simulink model "test_ffts"  (Simulink 6.2)
settings: Solver=ode45  StartTime=0.0  StopTime=300  RelTol=1e-3
undefined symbols (not defined in the file or in its folder): now
libraries: xbsIndex_r3 x1135, fft_library x1, simulink x1
(part 3 of 15)

== system test_ffts/r4_dit_fft ==
  a_in : Inport  Port=1  LatchInput=off
  b_in : Inport  Port=2  LatchInput=off
  c_in : Inport  Port=3  LatchInput=off
  d_in : Inport  Port=4  LatchInput=off
  sync_in : Inport  Port=5  LatchInput=off
  quadplex_bitrev : Subsystem  mask(Quadplex Bit Reverse Reorder){log2_size=4, n_bits=14}
      mask prompts: log2_size "Log2 Block Size"; n_bits "Number of Bits"
      mask help: Reorders the input sequences from normal order to bit reverse order (or vise versa).
      settings: AttributesFormatString=size = 16
      mask Help:
      | <pre>
      | Description::
      | 
      | Reorders the input sequences from normal order to bit reverse order (or vise versa).
      | 
      | Mask Parameters::
      | 
      | Log 2 Block Size (log2_size): The base-2 logarithm of the length of one complete input block.
      | This MUST be an integer because the current implementation requires that
      | the input block size MUST be a power of 2.  (aka "N")
      | 
      | Number of Bits (n_bits): Specifies the width of the real/imaginary components.
      | Width of each component is assumed equal.
      | </pre>
  quadplex_commutator : Subsystem  mask(Quadplex Commutator){log4_size=3, n_bits=14, use_bram=off}
      mask prompts: log4_size "Log4 Block Size"; n_bits "Bit Width"; use_bram "Use BRAM"
      mask help: The quadplex commutator performs a "quarter-blockwise" commutation of the four inputs. A "block" is 4^log4_size consecutive samples (i.e. always a power of 4). sync_in precedes the first data input sample by one clock cycle. Overall latency from sync_in to sync_out is 2^(log4_size)+2^(log4_size-1)+2.
      settings: AttributesFormatString=|
      | size = 64
      | 0/4 bram
      mask Help:
      | <pre>
      | Description::
      | 
      | The quadplex commutator performs a "quarter-blockwise" commutation of the four inputs.
      | A "block" is 4^log4_size consecutive samples (i.e. always a power of 4).
      | 
      | sync_in precedes the first data input sample by one clock cycle.
      | sync_out precedes the corresponding output sample by one clock cycle.
      | Overall latency from sync_in to sync_out is 2^(log4_size)+2^(log4_size-1)+2.
      | 
      | Mask Parameters::
      | 
      | Log4 Block Size (log4_size): The base-4 logarithm of the length of one complete input block.
      | This MUST be an integer because the current implementation requires that
      | the input block size MUST be a power of 4.  (aka "N")
      | 
      | Bit Width (n_bits): Specifies the width of the real/imaginary components.
      | Width of each component is assumed equal.
      | 
      | Use BRAM (use_bram): Check this checkbox to implement the internal delays using BRAM.
      | If unchecked, the internal delays will be implemented using SLR16 elements.
      | </pre>
  r4_dit_stage_1 : Subsystem  mask(Radix-4 DIT FFT Stage){n_stages=3, cur_stage=1, n_bits=8, bin_pt=7, shift=0, commutator_bram=off, twiddle_bram=off, n_bits_w=9, mult_latency=3, add_latency=1}
      mask prompts: n_stages "Total Stages (4^N points)"; cur_stage "Current Stage"; n_bits "Number of Bits In"; bin_pt "Binary Point In"; shift "Shift Bits"; commutator_bram "Use BRAM for Quadplex Commutator"; twiddle_bram "Use BRAM for Twiddle Coefficients"; n_bits_w "Twiddle Coefficient Bitwidth"; mult_latency "Multiplier Latency"; add_latency "Adder Latency"
      mask help: A radix-4 decimation-in-time Fast Fourier Transform stage.
      settings: AttributesFormatString=|
      | stage 1 of 3
      | delay slr
      | twiddle dist
      | shift 0
      mask Help:
      | <pre>
      | Description::
      | 
      | A radix-4 decimation-in-time Fast Fourier Transform stage.
      | 
      | This radix-4 decimation-in-time FFT stage is designed to be daisy chained together
      | to form a multi-stage FFT.  The resulting FFT will have (4^n_stages) points.
      | 
      | The four inputs to the chain are independent complex signals (e.g. A, B, C, and D).
      | 
      | The four outputs of the last stage of the chain are commuted such that the a_out signal is really
      | the first quarter of A's transform followed by the first quarter of B's transform, the first quarter
      | of C's transform and the first quarter of D's transform.  b_out is really the seconds quarter of
      | A's transform followed by the second quarter of B's transform and so on for the rest of b_out
      | as well as c_out and d_out.  Each quarter is in bit-reversed order.
      | 
      | If it is desired to have the four quarters of A's transform follow each other on the
      | same path (and so on for the transforms of B, C, and D), then a_out and b_out can
      | be fed through a quadplex_commutator with block size 4^n_stages.  This will result
      | in the four quarters of A's transform (or B's, C's, D's) being in sequential order,
      | but note that each quarter of A's transform will still remain in bit-reversed order
      | (i.e. each output is bit-reversed in quarterss; it is not bit reversed in its entirety).
      | 
      | The number of bits for each real and imaginary component grows by two through this stage.
      | If the input bit width is 17 or less, three embedded multipliers will be used per complex multiply.
      | If the input bit width is 18, four embedded multipliers will be used per complex multiply.
      | If the input bit width exceeds 18, then substantially more embedded multipliers will be used
      | per complex multiply.  Enabling "shifting" in some (or all) stages can limit the bit growth
      | to prevent this.
      | 
      | Mask Parameters::
      | 
      | Total Stages (n_stages):  The number of total stages in the FFT.
      | The FFT will have 4^n_stages points.
      | 
      | Current Stage (cur_stage):  The number of the current stage.  Note that stages are counted
      | from 1 to n_stages for DIT (i.e. cur_stage==1 for the first stage).
      | 
      | Number of Bits In (n_bits): Specifies the width of the real/imaginary components of ports
      | a_in and b_in.  Assumed equal for both components.  The real/imaginary components of
      | oorts a_out and b_out will be one bit wider.
      | 
      | Binary Point In (bin_pt): Specifies the binary point position of the real/imaginary
      | components of ports a_in and b_in.  Assumed equal for both components.
      | 
      | Shift Bits (shift): Specifies how many bits to shift (down) by.  A positive value causes
      | the specified number of least significant bits to be dropped.  Usually zero or positive values
      | are used to permit or limit bit growth, but negative values can be used to induce bit growth.
      | 
      | Use BRAM for Biplex Commutator (commutator_bram): Check this checkbox to implement
      | the biplex commutator using BRAM.  If unchecked, the biplex commutator will be implemented
      | using SLR16 elements (i.e. slices).
      | 
      | Use BRAM for Twiddle Coefficients (twiddle_bram): Check this checkbox to store twiddle
      | coefficients in BRAM.  If unchecked, the twiddle coefficients will be sored in distributed
      | memory (i.e. slices).
      | 
      | Twiddle Coefficient Bitwidth (n_bits_w): Specifies the width of the real/imaginary
      | components of the twiddle coefficients.  Assumed equal for both components.
      | 
      | Multiplier Latency (mult_latency): Latency to use for the underlying real multipliers.
      | 
      | Adder Latency (add_latency): Latency to use for the underlying real adders.
      | </pre>
  r4_dit_stage_2 : Subsystem  mask(Radix-4 DIT FFT Stage){n_stages=3, cur_stage=2, n_bits=10, bin_pt=7, shift=0, commutator_bram=off, twiddle_bram=off, n_bits_w=9, mult_latency=3, add_latency=1}
      mask prompts: n_stages "Total Stages (4^N points)"; cur_stage "Current Stage"; n_bits "Number of Bits In"; bin_pt "Binary Point In"; shift "Shift Bits"; commutator_bram "Use BRAM for Quadplex Commutator"; twiddle_bram "Use BRAM for Twiddle Coefficients"; n_bits_w "Twiddle Coefficient Bitwidth"; mult_latency "Multiplier Latency"; add_latency "Adder Latency"
      mask help: A radix-4 decimation-in-time Fast Fourier Transform stage.
      settings: AttributesFormatString=|
      | stage 2 of 3
      | delay slr
      | twiddle dist
      | shift 0
      mask Help:
      | <pre>
      | Description::
      | 
      | A radix-4 decimation-in-time Fast Fourier Transform stage.
      | 
      | This radix-4 decimation-in-time FFT stage is designed to be daisy chained together
      | to form a multi-stage FFT.  The resulting FFT will have (4^n_stages) points.
      | 
      | The four inputs to the chain are independent complex signals (e.g. A, B, C, and D).
      | 
      | The four outputs of the last stage of the chain are commuted such that the a_out signal is really
      | the first quarter of A's transform followed by the first quarter of B's transform, the first quarter
      | of C's transform and the first quarter of D's transform.  b_out is really the seconds quarter of
      | A's transform followed by the second quarter of B's transform and so on for the rest of b_out
      | as well as c_out and d_out.  Each quarter is in bit-reversed order.
      | 
      | If it is desired to have the four quarters of A's transform follow each other on the
      | same path (and so on for the transforms of B, C, and D), then a_out and b_out can
      | be fed through a quadplex_commutator with block size 4^n_stages.  This will result
      | in the four quarters of A's transform (or B's, C's, D's) being in sequential order,
      | but note that each quarter of A's transform will still remain in bit-reversed order
      | (i.e. each output is bit-reversed in quarterss; it is not bit reversed in its entirety).
      | 
      | The number of bits for each real and imaginary component grows by two through this stage.
      | If the input bit width is 17 or less, three embedded multipliers will be used per complex multiply.
      | If the input bit width is 18, four embedded multipliers will be used per complex multiply.
      | If the input bit width exceeds 18, then substantially more embedded multipliers will be used
      | per complex multiply.  Enabling "shifting" in some (or all) stages can limit the bit growth
      | to prevent this.
      | 
      | Mask Parameters::
      | 
      | Total Stages (n_stages):  The number of total stages in the FFT.
      | The FFT will have 4^n_stages points.
      | 
      | Current Stage (cur_stage):  The number of the current stage.  Note that stages are counted
      | from 1 to n_stages for DIT (i.e. cur_stage==1 for the first stage).
      | 
      | Number of Bits In (n_bits): Specifies the width of the real/imaginary components of ports
      | a_in and b_in.  Assumed equal for both components.  The real/imaginary components of
      | oorts a_out and b_out will be one bit wider.
      | 
      | Binary Point In (bin_pt): Specifies the binary point position of the real/imaginary
      | components of ports a_in and b_in.  Assumed equal for both components.
      | 
      | Shift Bits (shift): Specifies how many bits to shift (down) by.  A positive value causes
      | the specified number of least significant bits to be dropped.  Usually zero or positive values
      | are used to permit or limit bit growth, but negative values can be used to induce bit growth.
      | 
      | Use BRAM for Biplex Commutator (commutator_bram): Check this checkbox to implement
      | the biplex commutator using BRAM.  If unchecked, the biplex commutator will be implemented
      | using SLR16 elements (i.e. slices).
      | 
      | Use BRAM for Twiddle Coefficients (twiddle_bram): Check this checkbox to store twiddle
      | coefficients in BRAM.  If unchecked, the twiddle coefficients will be sored in distributed
      | memory (i.e. slices).
      | 
      | Twiddle Coefficient Bitwidth (n_bits_w): Specifies the width of the real/imaginary
      | components of the twiddle coefficients.  Assumed equal for both components.
      | 
      | Multiplier Latency (mult_latency): Latency to use for the underlying real multipliers.
      | 
      | Adder Latency (add_latency): Latency to use for the underlying real adders.
      | </pre>
  r4_dit_stage_3 : Subsystem  mask(Radix-4 DIT FFT Stage){n_stages=3, cur_stage=3, n_bits=12, bin_pt=7, shift=0, commutator_bram=off, twiddle_bram=off, n_bits_w=9, mult_latency=3, add_latency=1}
      mask prompts: n_stages "Total Stages (4^N points)"; cur_stage "Current Stage"; n_bits "Number of Bits In"; bin_pt "Binary Point In"; shift "Shift Bits"; commutator_bram "Use BRAM for Quadplex Commutator"; twiddle_bram "Use BRAM for Twiddle Coefficients"; n_bits_w "Twiddle Coefficient Bitwidth"; mult_latency "Multiplier Latency"; add_latency "Adder Latency"
      mask help: A radix-4 decimation-in-time Fast Fourier Transform stage.
      settings: AttributesFormatString=|
      | stage 3 of 3
      | delay slr
      | twiddle dist
      | shift 0
      mask Help:
      | <pre>
      | Description::
      | 
      | A radix-4 decimation-in-time Fast Fourier Transform stage.
      | 
      | This radix-4 decimation-in-time FFT stage is designed to be daisy chained together
      | to form a multi-stage FFT.  The resulting FFT will have (4^n_stages) points.
      | 
      | The four inputs to the chain are independent complex signals (e.g. A, B, C, and D).
      | 
      | The four outputs of the last stage of the chain are commuted such that the a_out signal is really
      | the first quarter of A's transform followed by the first quarter of B's transform, the first quarter
      | of C's transform and the first quarter of D's transform.  b_out is really the seconds quarter of
      | A's transform followed by the second quarter of B's transform and so on for the rest of b_out
      | as well as c_out and d_out.  Each quarter is in bit-reversed order.
      | 
      | If it is desired to have the four quarters of A's transform follow each other on the
      | same path (and so on for the transforms of B, C, and D), then a_out and b_out can
      | be fed through a quadplex_commutator with block size 4^n_stages.  This will result
      | in the four quarters of A's transform (or B's, C's, D's) being in sequential order,
      | but note that each quarter of A's transform will still remain in bit-reversed order
      | (i.e. each output is bit-reversed in quarterss; it is not bit reversed in its entirety).
      | 
      | The number of bits for each real and imaginary component grows by two through this stage.
      | If the input bit width is 17 or less, three embedded multipliers will be used per complex multiply.
      | If the input bit width is 18, four embedded multipliers will be used per complex multiply.
      | If the input bit width exceeds 18, then substantially more embedded multipliers will be used
      | per complex multiply.  Enabling "shifting" in some (or all) stages can limit the bit growth
      | to prevent this.
      | 
      | Mask Parameters::
      | 
      | Total Stages (n_stages):  The number of total stages in the FFT.
      | The FFT will have 4^n_stages points.
      | 
      | Current Stage (cur_stage):  The number of the current stage.  Note that stages are counted
      | from 1 to n_stages for DIT (i.e. cur_stage==1 for the first stage).
      | 
      | Number of Bits In (n_bits): Specifies the width of the real/imaginary components of ports
      | a_in and b_in.  Assumed equal for both components.  The real/imaginary components of
      | oorts a_out and b_out will be one bit wider.
      | 
      | Binary Point In (bin_pt): Specifies the binary point position of the real/imaginary
      | components of ports a_in and b_in.  Assumed equal for both components.
      | 
      | Shift Bits (shift): Specifies how many bits to shift (down) by.  A positive value causes
      | the specified number of least significant bits to be dropped.  Usually zero or positive values
      | are used to permit or limit bit growth, but negative values can be used to induce bit growth.
      | 
      | Use BRAM for Biplex Commutator (commutator_bram): Check this checkbox to implement
      | the biplex commutator using BRAM.  If unchecked, the biplex commutator will be implemented
      | using SLR16 elements (i.e. slices).
      | 
      | Use BRAM for Twiddle Coefficients (twiddle_bram): Check this checkbox to store twiddle
      | coefficients in BRAM.  If unchecked, the twiddle coefficients will be sored in distributed
      | memory (i.e. slices).
      | 
      | Twiddle Coefficient Bitwidth (n_bits_w): Specifies the width of the real/imaginary
      | components of the twiddle coefficients.  Assumed equal for both components.
      | 
      | Multiplier Latency (mult_latency): Latency to use for the underlying real multipliers.
      | 
      | Adder Latency (add_latency): Latency to use for the underlying real adders.
      | </pre>
  a_out : Outport
  b_out : Outport  Port=2
  c_out : Outport  Port=3
  d_out : Outport  Port=4
  sync_out : Outport  Port=5
  wires:
  a_in/1 -> r4_dit_stage_1/1(a_in)
  b_in/1 -> r4_dit_stage_1/2(b_in)
  c_in/1 -> r4_dit_stage_1/3(c_in)
  d_in/1 -> r4_dit_stage_1/4(d_in)
  sync_in/1 -> r4_dit_stage_1/5(sync_in)
  r4_dit_stage_1/1(a_out) -> r4_dit_stage_2/1(a_in)
  r4_dit_stage_1/2(b_out) -> r4_dit_stage_2/2(b_in)
  r4_dit_stage_1/3(c_out) -> r4_dit_stage_2/3(c_in)
  r4_dit_stage_1/4(d_out) -> r4_dit_stage_2/4(d_in)
  r4_dit_stage_1/5(sync_out) -> r4_dit_stage_2/5(sync_in)
  r4_dit_stage_2/1(a_out) -> r4_dit_stage_3/1(a_in)
  r4_dit_stage_2/2(b_out) -> r4_dit_stage_3/2(b_in)
  r4_dit_stage_2/3(c_out) -> r4_dit_stage_3/3(c_in)
  r4_dit_stage_2/4(d_out) -> r4_dit_stage_3/4(d_in)
  r4_dit_stage_2/5(sync_out) -> r4_dit_stage_3/5(sync_in)
  r4_dit_stage_3/1(a_out) -> quadplex_commutator/1(a)
  r4_dit_stage_3/3(c_out) -> quadplex_commutator/2(b)
  r4_dit_stage_3/2(b_out) -> quadplex_commutator/3(c)
  r4_dit_stage_3/4(d_out) -> quadplex_commutator/4(d)
  r4_dit_stage_3/5(sync_out) -> quadplex_commutator/5(sync_in)
  quadplex_commutator/1(abcd0) -> quadplex_bitrev/1(a_in)
  quadplex_commutator/2(abcd1) -> quadplex_bitrev/2(b_in)
  quadplex_commutator/3(abcd2) -> quadplex_bitrev/3(c_in)
  quadplex_commutator/4(abcd3) -> quadplex_bitrev/4(d_in)
  quadplex_commutator/5(sync_out) -> quadplex_bitrev/5(sync_in)
  quadplex_bitrev/1(a_out) -> a_out/1
  quadplex_bitrev/2(b_out) -> b_out/1
  quadplex_bitrev/3(c_out) -> c_out/1
  quadplex_bitrev/4(d_out) -> d_out/1
  quadplex_bitrev/5(sync_out) -> sync_out/1

== system test_ffts/ri_to_c ==
  re : Inport  Port=1  LatchInput=off
  im : Inport  Port=2  LatchInput=off
  concat : xbsIndex_r3/Concat  num_inputs=2  explicit_period=off  period=1  dbl_ovrd=off
  force_im : xbsIndex_r3/Reinterpret  force_arith_type=on  arith_type=Unsigned  force_bin_pt=on  bin_pt=0  force_valid=on
  force_re : xbsIndex_r3/Reinterpret  force_arith_type=on  arith_type=Unsigned  force_bin_pt=on  bin_pt=0  force_valid=on
  c : Outport
  wires:
  force_re/1 -> concat/1
  force_im/1 -> concat/2
  re/1 -> force_re/1
  concat/1 -> c/1
  im/1 -> force_im/1

== system test_ffts/ri_to_c1 ==
  re : Inport  Port=1  LatchInput=off
  im : Inport  Port=2  LatchInput=off
  concat : xbsIndex_r3/Concat  num_inputs=2  explicit_period=off  period=1  dbl_ovrd=off
  force_im : xbsIndex_r3/Reinterpret  force_arith_type=on  arith_type=Unsigned  force_bin_pt=on  bin_pt=0  force_valid=on
  force_re : xbsIndex_r3/Reinterpret  force_arith_type=on  arith_type=Unsigned  force_bin_pt=on  bin_pt=0  force_valid=on
  c : Outport
  wires:
  im/1 -> force_im/1
  concat/1 -> c/1
  re/1 -> force_re/1
  force_im/1 -> concat/2
  force_re/1 -> concat/1

== system test_ffts/ri_to_c2 ==
  re : Inport  Port=1  LatchInput=off
  im : Inport  Port=2  LatchInput=off
  concat : xbsIndex_r3/Concat  num_inputs=2  explicit_period=off  period=1  dbl_ovrd=off
  force_im : xbsIndex_r3/Reinterpret  force_arith_type=on  arith_type=Unsigned  force_bin_pt=on  bin_pt=0  force_valid=on
  force_re : xbsIndex_r3/Reinterpret  force_arith_type=on  arith_type=Unsigned  force_bin_pt=on  bin_pt=0  force_valid=on
  c : Outport
  wires:
  im/1 -> force_im/1
  concat/1 -> c/1
  re/1 -> force_re/1
  force_im/1 -> concat/2
  force_re/1 -> concat/1

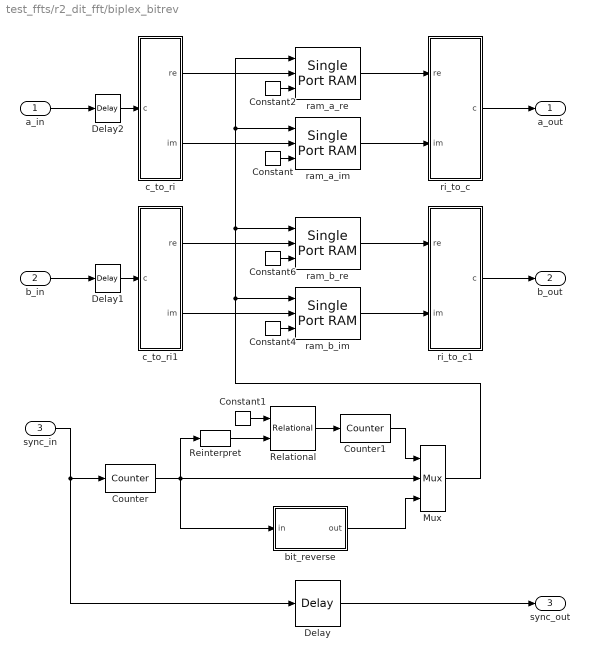
== system test_ffts/r2_dit_fft/biplex_bitrev ==
  a_in : Inport  Port=1  LatchInput=off
  b_in : Inport  Port=2  LatchInput=off
  sync_in : Inport  Port=3  LatchInput=off
  Constant{,2,4,6} (4 alike) : xbsIndex_r3/Constant  const=1  equ=P=C  arith_type=Boolean  n_bits=1  bin_pt=0  opselect=C  inp2=PCIN>>17  opr=+  inp1=P  carry=CIN  iostate=0  explicit_period=on  period=1  dbl_ovrd=off
  Constant1 : xbsIndex_r3/Constant  const=-1  equ=P=C  arith_type="Signed  (2's comp)"  n_bits=1  bin_pt=0  opselect=C  inp2=PCIN>>17  opr=+  inp1=P  carry=CIN  iostate=0  explicit_period=on  period=1  dbl_ovrd=off
  Counter : xbsIndex_r3/Counter  cnt_type=Free Running  n_bits=5  bin_pt=0  arith_type=Unsigned  start_count=0  cnt_to=Inf  cnt_by_val=1  operation=Up  explicit_period=off  period=1  load_pin=off  rst=on  en=off  dbl_ovrd=off  show_param=off  use_rpm=on  gen_core=off
      settings: xl_area=[0, 0, 0, 0, 0, 0, 0]
  Counter1 : xbsIndex_r3/Counter  cnt_type=Free Running  n_bits=1  bin_pt=0  arith_type=Unsigned  start_count=0  cnt_to=Inf  cnt_by_val=1  operation=Up  explicit_period=off  period=1  load_pin=off  rst=off  en=on  dbl_ovrd=off  show_param=off  use_rpm=on  gen_core=off
      settings: xl_area=[0, 0, 0, 0, 0, 0, 0]
  Delay : xbsIndex_r3/Delay  latency=34  reg_retiming=off  explicit_period=off  period=1  en=off  accept_only_valid=off  init_zero=on  dbl_ovrd=off  show_param=off
      settings: xl_area=[0, 0, 0, 0, 0, 0, 0]
  Delay1 : xbsIndex_r3/Delay  latency=1  reg_retiming=off  explicit_period=off  period=1  en=off  accept_only_valid=off  init_zero=on  dbl_ovrd=off  show_param=off
      settings: xl_area=[0, 0, 0, 0, 0, 0, 0]
  Delay2 : xbsIndex_r3/Delay  latency=1  reg_retiming=off  explicit_period=off  period=1  en=off  accept_only_valid=off  init_zero=on  dbl_ovrd=off  show_param=off
      settings: xl_area=[0, 0, 0, 0, 0, 0, 0]
  Mux : xbsIndex_r3/Mux  inputs=2  precision=Full  arith_type="Signed  (2's comp)"  n_bits=8  bin_pt=2  quantization=Truncate  overflow=Wrap  latency=1  explicit_period=off  period=1  en=off  dbl_ovrd=off  show_param=off  mux_type=off  use_rpm=off  gen_core=off
      settings: xl_area=[0, 0, 0, 0, 0, 0, 0]
  Reinterpret : xbsIndex_r3/Reinterpret  force_arith_type=on  arith_type="Signed  (2's comp)"  force_bin_pt=off  bin_pt=0  force_valid=on
  Relational : xbsIndex_r3/Relational  mode=a=b  latency=1  explicit_period=off  period=1  en=off  dbl_ovrd=off  show_param=off
      settings: xl_area=[0, 0, 0, 0, 0, 0, 0]
  bit_reverse : Subsystem  mask(Bit Reversal){n_bits=5}
      mask prompts: n_bits "Number of Bits"
      mask help: Reverses the bit order of the input. Input must be unsigned with binary point at position 0. Costs nothing in hardware.
      settings: AttributesFormatString=5 bits
      mask Help:
      | <pre>
      | Description::
      | 
      | Reverses the bit order of the input.
      | 
      | Input must be unsigned with binary point at position 0.
      | 
      | Costs nothing in hardware.
      | 
      | Mask Parameters::
      | 
      | Number of Bits (n_bits): Specifies the width of the input.
      | </pre>
  c_to_ri : Subsystem  mask(Complex to Real-Imag){n_bits=14, bin_pt=0}
      mask prompts: n_bits "Bit Width"; bin_pt "Binary Point"
      mask help: Outputs real and imaginary components of a complex input.
      settings: AttributesFormatString=14_0 r/i
      mask Help:
      | <pre>
      | Description::
      | 
      | Outputs real and imaginary components of a complex input.
      | Useful for simplifying interconnects.
      | See also: Real-Imag to Complex (ri_to_c)
      | 
      | Mask Parameters::
      | 
      | Bit Width (n_bits): Specifies the width of the real/imaginary components.
      | Assumed equal for both components.
      | 
      | Binary Point (bin_pt): Specifies the binary point location in the real/imaginary components.
      | Assumed equal for both components.
      | </pre>
  c_to_ri1 : Subsystem  mask(Complex to Real-Imag){n_bits=14, bin_pt=0}
      mask prompts: n_bits "Bit Width"; bin_pt "Binary Point"
      mask help: Outputs real and imaginary components of a complex input.
      settings: AttributesFormatString=14_0 r/i
      mask Help:
      | <pre>
      | Description::
      | 
      | Outputs real and imaginary components of a complex input.
      | Useful for simplifying interconnects.
      | See also: Real-Imag to Complex (ri_to_c)
      | 
      | Mask Parameters::
      | 
      | Bit Width (n_bits): Specifies the width of the real/imaginary components.
      | Assumed equal for both components.
      | 
      | Binary Point (bin_pt): Specifies the binary point location in the real/imaginary components.
      | Assumed equal for both components.
      | </pre>
  ram_a_im : xbsIndex_r3/Single Port RAM  depth=32  initVector=0  write_mode=Read Before Write  latency=1  init_zero=on  explicit_period=off  period=1  rst=off  init_reg=0  en=off  dbl_ovrd=off  show_param=on  distributed_mem=off  use_rpm=off  gen_core=off
      settings: xl_area=[0, 0, 0, 0, 0, 0, 0]
  ram_a_re : xbsIndex_r3/Single Port RAM  depth=32  initVector=0  write_mode=Read Before Write  latency=1  init_zero=on  explicit_period=off  period=1  rst=off  init_reg=0  en=off  dbl_ovrd=off  show_param=on  distributed_mem=off  use_rpm=off  gen_core=off
      settings: xl_area=[0, 0, 0, 0, 0, 0, 0]
  ram_b_im : xbsIndex_r3/Single Port RAM  depth=32  initVector=0  write_mode=Read Before Write  latency=1  init_zero=on  explicit_period=off  period=1  rst=off  init_reg=0  en=off  dbl_ovrd=off  show_param=on  distributed_mem=off  use_rpm=off  gen_core=off
      settings: xl_area=[0, 0, 0, 0, 0, 0, 0]
  ram_b_re : xbsIndex_r3/Single Port RAM  depth=32  initVector=0  write_mode=Read Before Write  latency=1  init_zero=on  explicit_period=off  period=1  rst=off  init_reg=0  en=off  dbl_ovrd=off  show_param=on  distributed_mem=off  use_rpm=off  gen_core=off
      settings: xl_area=[0, 0, 0, 0, 0, 0, 0]
  ri_to_c : Subsystem
      mask Type: Real-Imag to Complex
      mask Description: Concatenates real and imaginary inputs into a complex output.
      mask Help:
      | <pre>
      | Description::
      | 
      | Concatenates a real and imaginary input into a complex output.
      | Useful for simplifying interconnects.
      | See also: Complex to Real-Imag (c_to_ri)
      | 
      | Mask Parameters::
      | 
      | (N/A)
      | </pre>
  ri_to_c1 : Subsystem
      mask Type: Real-Imag to Complex
      mask Description: Concatenates real and imaginary inputs into a complex output.
      mask Help:
      | <pre>
      | Description::
      | 
      | Concatenates a real and imaginary input into a complex output.
      | Useful for simplifying interconnects.
      | See also: Complex to Real-Imag (c_to_ri)
      | 
      | Mask Parameters::
      | 
      | (N/A)
      | </pre>
  a_out : Outport
  b_out : Outport  Port=2
  sync_out : Outport  Port=3
  wires:
  Reinterpret/1 -> Relational/2
  Relational/1 -> Counter1/1
  Constant1/1 -> Relational/1
  Counter1/1 -> Mux/1
  Counter/1 -> Reinterpret/1, Mux/2, bit_reverse/1(in)
  Constant6/1 -> ram_b_re/3
  Constant4/1 -> ram_b_im/3
  Constant2/1 -> ram_a_re/3
  Constant/1 -> ram_a_im/3
  Delay/1 -> sync_out/1
  Mux/1 -> ram_b_im/1, ram_b_re/1, ram_a_im/1, ram_a_re/1
  bit_reverse/1(out) -> Mux/3
  b_in/1 -> Delay1/1
  a_in/1 -> Delay2/1
  c_to_ri1/2(im) -> ram_b_im/2
  c_to_ri1/1(re) -> ram_b_re/2
  c_to_ri/2(im) -> ram_a_im/2
  c_to_ri/1(re) -> ram_a_re/2
  ri_to_c1/1(c) -> b_out/1
  ri_to_c/1(c) -> a_out/1
  ram_b_im/1 -> ri_to_c1/2(im)
  ram_b_re/1 -> ri_to_c1/1(re)
  ram_a_im/1 -> ri_to_c/2(im)
  ram_a_re/1 -> ri_to_c/1(re)
  sync_in/1 -> Delay/1, Counter/1
  Delay1/1 -> c_to_ri1/1(c)
  Delay2/1 -> c_to_ri/1(c)

== system test_ffts/r2_dit_fft/biplex_commutator ==
  AloAhi : Inport  Port=1  LatchInput=off
  BloBhi : Inport  Port=2  LatchInput=off
  sync_in : Inport  Port=3  LatchInput=off
  Counter : xbsIndex_r3/Counter  cnt_type=Free Running  n_bits=6  bin_pt=0  arith_type=Unsigned  start_count=0  cnt_to=Inf  cnt_by_val=1  operation=Up  explicit_period=off  period=1  load_pin=off  rst=on  en=off  dbl_ovrd=off  show_param=off  use_rpm=on  gen_core=off
      settings: xl_area=[0, 0, 0, 0, 0, 0, 0]
  Delay : xbsIndex_r3/Delay  latency=33  reg_retiming=off  explicit_period=off  period=1  en=off  accept_only_valid=off  init_zero=on  dbl_ovrd=off  show_param=off
      settings: xl_area=[0, 0, 0, 0, 0, 0, 0]
  Mux : xbsIndex_r3/Mux  inputs=2  precision=Full  arith_type="Signed  (2's comp)"  n_bits=8  bin_pt=2  quantization=Truncate  overflow=Wrap  latency=1  explicit_period=off  period=1  en=off  dbl_ovrd=off  show_param=off  mux_type=off  use_rpm=off  gen_core=off
      settings: xl_area=[0, 0, 0, 0, 0, 0, 0]
  Mux1 : xbsIndex_r3/Mux  inputs=2  precision=Full  arith_type="Signed  (2's comp)"  n_bits=8  bin_pt=2  quantization=Truncate  overflow=Wrap  latency=1  explicit_period=off  period=1  en=off  dbl_ovrd=off  show_param=on  mux_type=off  use_rpm=off  gen_core=off
      settings: xl_area=[0, 0, 0, 0, 0, 0, 0]
  delay_b : Subsystem  mask(Complex Delay){delay_depth=32, n_bits=14, use_bram=on}
      mask prompts: delay_depth "Delay Depth"; n_bits "Bit Width"; use_bram "Use BRAM"
      mask help: A delay block that treats its input as complex, splits it into real and imaginary components, delays each component by a specified amount, and then re-joins them into a complex output. The underlying storage is user-selectable (either BRAM or SLR16 elements).
      settings: AttributesFormatString=|
      | depth = 32
      | delay bram
      mask Help:
      | <pre>
      | Description::
      | 
      | A delay block that treats its input as complex, splits it into real and imaginary components,
      | delays each component by a specified amount, and then re-joins them into a complex
      | output.  The underlying storage is user-selectable (either BRAM or SLR16 elements).
      | 
      | Mask Parameters::
      | 
      | Delay Depth (delay_depth): The length of the delay.
      | 
      | Bit Width (n_bits): Specifies the width of the real/imaginary components.
      | Width of each component is assumed equal.
      | 
      | Use BRAM (use_bram): Check this checkbox to implement the delay using BRAM.
      | If unchecked, the delay will be implemented using SLR16 elements.
      | </pre>
  delay_lo : Subsystem  mask(Complex Delay){delay_depth=32, n_bits=14, use_bram=on}
      mask prompts: delay_depth "Delay Depth"; n_bits "Bit Width"; use_bram "Use BRAM"
      mask help: A delay block that treats its input as complex, splits it into real and imaginary components, delays each component by a specified amount, and then re-joins them into a complex output. The underlying storage is user-selectable (either BRAM or SLR16 elements).
      settings: AttributesFormatString=|
      | depth = 32
      | delay bram
      mask Help:
      | <pre>
      | Description::
      | 
      | A delay block that treats its input as complex, splits it into real and imaginary components,
      | delays each component by a specified amount, and then re-joins them into a complex
      | output.  The underlying storage is user-selectable (either BRAM or SLR16 elements).
      | 
      | Mask Parameters::
      | 
      | Delay Depth (delay_depth): The length of the delay.
      | 
      | Bit Width (n_bits): Specifies the width of the real/imaginary components.
      | Width of each component is assumed equal.
      | 
      | Use BRAM (use_bram): Check this checkbox to implement the delay using BRAM.
      | If unchecked, the delay will be implemented using SLR16 elements.
      | </pre>
  top_bit : xbsIndex_r3/Slice  mode=Upper Bit Location + Width  nbits=1  bit1=0  base1=MSB of Input  bit0=0  base0=LSB of Input  boolean_output=off  explicit_period=off  period=1  dbl_ovrd=off
  AloBlo : Outport
  AhiBhi : Outport  Port=2
  sync_out : Outport  Port=3
  wires:
  Delay/1 -> sync_out/1
  delay_lo/1(out) -> AloBlo/1
  Mux/1 -> delay_lo/1(in)
  delay_b/1(out) -> Mux/3, Mux1/2
  BloBhi/1 -> delay_b/1(in)
  Mux1/1 -> AhiBhi/1
  AloAhi/1 -> Mux1/3, Mux/2
  top_bit/1 -> Mux/1, Mux1/1
  Counter/1 -> top_bit/1
  sync_in/1 -> Delay/1, Counter/1

== system test_ffts/r2_dit_fft/r2_dit_stage_1 ==
  a_in : Inport  Port=1  LatchInput=off
  b_in : Inport  Port=2  LatchInput=off
  sync_in : Inport  Port=3  LatchInput=off
  biplex_commutator : Subsystem  mask(Biplex Commutator){log2_size=6, n_bits=8, use_bram=off}
      mask prompts: log2_size "Log2 Block Size"; n_bits "Bit Width"; use_bram "Use BRAM"
      mask help: The biplex commutator commutes the first half of the BloBhi input "block" with the last half of the AloAhi input "block". A "block" is 2^log2_size consecutive samples (i.e. always a power of 2). sync_in precedes the first data input sample by one clock cycle. Overall latency from sync_in to sync_out is 2^(log2_size-1)+1.
      settings: AttributesFormatString=|
      | size = 64
      | delay slr
      mask Help:
      | <pre>
      | Description::
      | 
      | The biplex commutator commutes the first half of the BloBhi input "block"  with the last half
      | of the AloAhi input "block".  A "block" is 2^log2_size consecutive samples (i.e. always a
      | power of 2).
      | 
      | sync_in precedes the first data input sample by one clock cycle.
      | sync_out precedes the corresponding output sample by one clock cycle.
      | Overall latency from sync_in to sync_out is 2^(N-1)+1.
      | 
      | Mask Parameters::
      | 
      | Log 2 Block Size (log2_size): The base-2 logarithm of the length of one complete input block.
      | This MUST be an integer because the current implementation requires that
      | the input block size MUST be a power of 2.  (aka "N")
      | 
      | Bit Width (n_bits): Specifies the width of the real/imaginary components.
      | Width of each component is assumed equal.
      | 
      | Use BRAM (use_bram): Check this checkbox to implement the internal delays using BRAM.
      | If unchecked, the internal delays will be implemented using SLR16 elements.
      | </pre>
  r2_butterfly : Subsystem  mask(Radix-2 Butterfly){n_bits=8, shift=0, quantization=Truncate, add_latency=1}
      mask prompts: n_bits "Bit Width In"; shift "Shift Bits"; add_latency "Adder Latency"
      mask help: The radix-2 butterfly produces a+b and a-b outputs for a and b inputs.
      settings: AttributesFormatString=shift 0
      mask Help:
      | <pre>
      | Description::
      | 
      | The radix-2 butterfly produces a+b and a-b outputs for a and b inputs.
      | The outputs are one bit wider than the inputs.
      | The output precision (i.e. the number of fractional bits) stays the same.
      | 
      | Mask Parameters::
      | 
      | Bit Width In (n_bits): Specifies the width of the real/imaginary components.
      | Width of each component is assumed equal.
      | 
      | Shift Bits (shift): Specifies how many bits to shift (down) by.  A positive value causes
      | the specified number of least significant bits to be dropped.  Usually zero or positive values
      | are used to permit or limit bit growth, but negative values can be used to induce bit growth.
      | 
      | Quantization (quantization): Specifies quantization handling (when shift bits > 0).
      | 
      | Adder Latency (add_latency): Latency to use for the underlying real adders.
      | </pre>
      mask StyleString: edit,edit,popup(Truncate|Round  (unbiased: +/- Inf)|Round  (unbiased: Even Values)),edit
  r2_twiddle : Subsystem
      mask Type: Radix-2 Stage-1 Twiddle Stage
      mask Description: A stage-1 twiddle stage for radix-2 Fast Fourier Transforms. Since there are no twiddles in stage 1 of an FFT, this is just a dummy placeholder block that passes its inputs through to its outputs.    Since it is a no-op, its use is completely optional.
      mask Help:
      | <pre>
      | Description::
      | 
      | A stage-1 twiddle stage for radix-2 Fast Fourier Transforms.
      | 
      | Since there are no twiddles in stage 1 of an FFT, this is just a dummy placeholder
      | block that passes its inputs through to its outputs.
      | 
      | Since it is a no-op, its use is completely optional.
      | 
      | Note that stages are counted from 1 to n_stages for DIT (i.e. cur_stage==1 for the first stage)
      | and n_stages to 1for DIF (i.e. cur_stage==1 for the last stage).  Therefore, this block, if used,
      | should be the first twiddle stage of a DIT FFT or the last twiddle stage of a DIF FFT.
      | 
      | Mask Parameters::
      | 
      | (N/A)
  a_out : Outport
  b_out : Outport  Port=2
  sync_out : Outport  Port=3
  wires:
  r2_butterfly/3(sync_out) -> sync_out/1
  r2_butterfly/2(a-b) -> b_out/1
  r2_butterfly/1(a+b) -> a_out/1
  sync_in/1 -> biplex_commutator/3(sync_in)
  b_in/1 -> biplex_commutator/2(BloBhi)
  a_in/1 -> biplex_commutator/1(AloAhi)
  biplex_commutator/3(sync_out) -> r2_twiddle/3(sync_in)
  biplex_commutator/2(AhiBhi) -> r2_twiddle/2(b_in)
  biplex_commutator/1(AloBlo) -> r2_twiddle/1(a_in)
  r2_twiddle/1(a_out) -> r2_butterfly/1(a)
  r2_twiddle/2(b_out) -> r2_butterfly/2(b)
  r2_twiddle/3(sync_out) -> r2_butterfly/3(sync_in)

== system test_ffts/r2_dit_fft/r2_dit_stage_2 ==
  a_in : Inport  Port=1  LatchInput=off
  b_in : Inport  Port=2  LatchInput=off
  sync_in : Inport  Port=3  LatchInput=off
  biplex_commutator : Subsystem  mask(Biplex Commutator){log2_size=5, n_bits=9, use_bram=off}
      mask prompts: log2_size "Log2 Block Size"; n_bits "Bit Width"; use_bram "Use BRAM"
      mask help: The biplex commutator commutes the first half of the BloBhi input "block" with the last half of the AloAhi input "block". A "block" is 2^log2_size consecutive samples (i.e. always a power of 2). sync_in precedes the first data input sample by one clock cycle. Overall latency from sync_in to sync_out is 2^(log2_size-1)+1.
      settings: AttributesFormatString=|
      | size = 32
      | delay slr
      mask Help:
      | <pre>
      | Description::
      | 
      | The biplex commutator commutes the first half of the BloBhi input "block"  with the last half
      | of the AloAhi input "block".  A "block" is 2^log2_size consecutive samples (i.e. always a
      | power of 2).
      | 
      | sync_in precedes the first data input sample by one clock cycle.
      | sync_out precedes the corresponding output sample by one clock cycle.
      | Overall latency from sync_in to sync_out is 2^(N-1)+1.
      | 
      | Mask Parameters::
      | 
      | Log 2 Block Size (log2_size): The base-2 logarithm of the length of one complete input block.
      | This MUST be an integer because the current implementation requires that
      | the input block size MUST be a power of 2.  (aka "N")
      | 
      | Bit Width (n_bits): Specifies the width of the real/imaginary components.
      | Width of each component is assumed equal.
      | 
      | Use BRAM (use_bram): Check this checkbox to implement the internal delays using BRAM.
      | If unchecked, the internal delays will be implemented using SLR16 elements.
      | </pre>
  r2_butterfly : Subsystem  mask(Radix-2 Butterfly with optional -j twiddle (DIT, twiddle before butterfly)){n_bits=9, shift=0, quantization=Truncate, add_latency=1}
      mask prompts: n_bits "Bit Width In"; shift "Shift Bits"; add_latency "Adder Latency"
      mask help: The radix-2 butterfly produces a+b and a-b outputs for a and b inputs. This variation efficiently includes an optional -j twiddle factor that can be applied before the butterfly (suitable for use in stage two of a DIT FFT).
      settings: AttributesFormatString=shift 0
      mask Help:
      | <pre>
      | Description::
      | 
      | The radix-2 butterfly produces a+b and a-b outputs for a and b inputs.
      | This variation efficiently includes an optional -j twiddle factor that can be
      | applied before the butterfly (suitable for use in stage two of a DIT FFT).
      | 
      | The -j twiddle factor is applied to tbe b input when tw_en is high,
      | thus producing a-jb on the a+b output and a+jb on the a-b output.
      | 
      | The outputs are one bit wider than the inputs.
      | The output precision (i.e. the number of fractional bits) stays the same.
      | 
      | Mask Parameters::
      | 
      | Bit Width In (n_bits): Specifies the width of the real/imaginary components.
      | Width of each component is assumed equal.
      | 
      | Shift Bits (shift): Specifies how many bits to shift (down) by.  A positive value causes
      | the specified number of least significant bits to be dropped.  Usually zero or positive values
      | are used to permit or limit bit growth, but negative values can be used to induce bit growth.
      | 
      | Quantization (quantization): Specifies quantization handling (when shift bits > 0).
      | 
      | Adder Latency (add_latency): Latency to use for the underlying real adders.
      | </pre>
      mask StyleString: edit,edit,popup(Truncate|Round  (unbiased: +/- Inf)|Round  (unbiased: Even Values)),edit
  r2_twiddle : Subsystem  mask(Radix-2 DIT Stage-2 Twiddle Stage){n_stages=6}
      mask prompts: n_stages "Total Stages"
      mask help: A stage-2 twiddle stage for radix-2 Decimation in Time Fast Fourier Transforms. The FFT is assumed to have inputs in normal order and outputs in bit-reversed order. This block must be used in conjuction with an r2_butterfly_dit_j_opt block (or equivalent) which has an optional -j twiddle factor built in.
      mask Help:
      | <pre>
      | Description::
      | 
      | A stage-2 twiddle stage for radix-2 Decimation in Time Fast Fourier Transforms.
      | 
      | The FFT is assumed to have inputs in normal order and outputs in bit-reversed order.
      | 
      | This block must be used in conjuction with an r2_butterfly_dit_j_opt block (or equivalent)
      | which has an optional -j twiddle factor built in.  This block does no twidlling at all; it just provides
      | a tw_en output for use with an r2_butterfly_dit_j_opt block (or equivalent).
      | 
      | Mask Parameters::
      | 
      | Total Stages (n_stages):  The number of total stages in the FFT.
      | The FFT will have 2^n_stages points.
  a_out : Outport
  b_out : Outport  Port=2
  sync_out : Outport  Port=3
  wires:
  r2_butterfly/3(sync_out) -> sync_out/1
  r2_butterfly/2(a-b) -> b_out/1
  r2_butterfly/1(a+b) -> a_out/1
  sync_in/1 -> biplex_commutator/3(sync_in)
  b_in/1 -> biplex_commutator/2(BloBhi)
  a_in/1 -> biplex_commutator/1(AloAhi)
  biplex_commutator/3(sync_out) -> r2_twiddle/3(sync_in)
  biplex_commutator/2(AhiBhi) -> r2_twiddle/2(b_in)
  biplex_commutator/1(AloBlo) -> r2_twiddle/1(a_in)
  r2_twiddle/1(a_out) -> r2_butterfly/1(a)
  r2_twiddle/2(b_out) -> r2_butterfly/2(b)
  r2_twiddle/3(sync_out) -> r2_butterfly/3(sync_in)
  r2_twiddle/4(tw_en) -> r2_butterfly/4(tw_en)
